simulink model "Math_transpose"  (R2017b)
settings: Solver=FixedStepDiscrete  StartTime=0.0  StopTime=10.0  FixedStep=0.200000  RelTol=1e-3  EnableMultiTasking=on
model workspace (MAT data in the model file):
  already_pp = 0
settings Model: Creator=ktrinh  LastModifiedBy=hbourbou
settings OptimizationCC: LifeSpan=inf
settings DebuggingCC: AlgebraicLoopMsg=error  ArtificialAlgebraicLoopMsg=error  SFUnexpectedBacktrackingDiag=warning  SFNoUnconditionalDefaultTransitionDiag=warning  SFExecutionAtInitializationDiag=none
settings HardwareCC: ProdBitPerSizeT=32  ProdBitPerPtrDiffT=32  ProdWordSize=32  ProdHWDeviceType=Specified
settings CodeAppCC: StateflowObjectComments=on
settings GRTTargetCC: TargetLangStandard=C89/C90 (ANSI)  GeneratePreprocessorConditionals=Disable all
settings ConfigComp: CovMetricSettings=dw  CovHtmlReporting=on  CovSaveCumulativeToWorkspaceVar=on  CovSaveSingleToWorkspaceVar=on  CovExternalEMLEnable=off

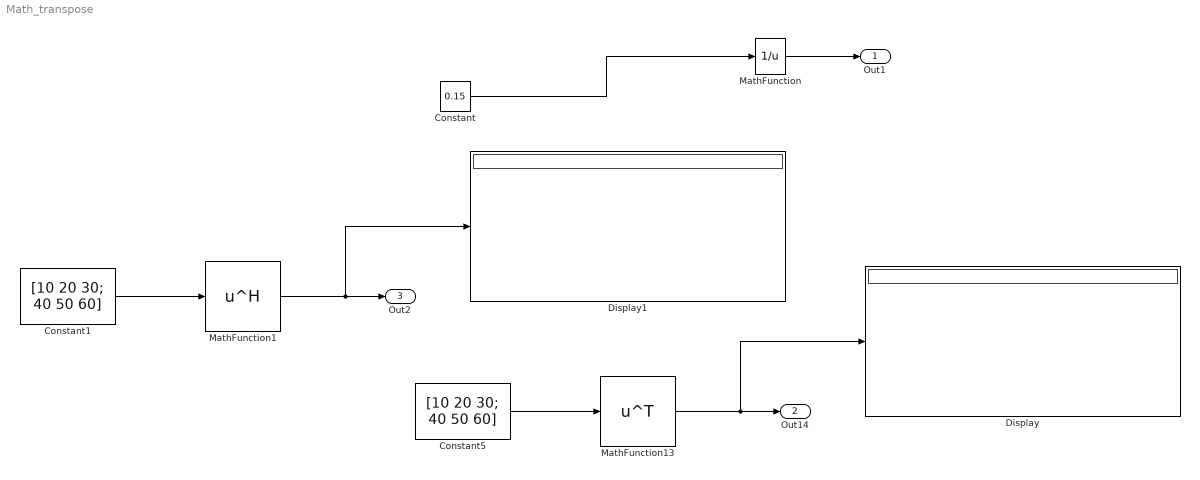
== system Math_transpose ==
  Constant : Constant  Value=0.15
  Constant1 : Constant  Value=[10 20 30; 40 50 60]
  Constant5 : Constant  Value=[10 20 30; 40 50 60]
  Display : Display
  Display1 : Display
  MathFunction : Math  Operator=reciprocal  SaturateOnIntegerOverflow=on
  MathFunction1 : Math  Operator=hermitian  SaturateOnIntegerOverflow=on
  MathFunction13 : Math  Operator=transpose  SaturateOnIntegerOverflow=on
  Out1 : Outport
  Out14 : Outport  Port=2
  Out2 : Outport  Port=3
  wires:
  MathFunction/1 -> Out1/1
  Constant/1 -> MathFunction/1
  MathFunction13/1 -> Display/1, Out14/1
  Constant5/1 -> MathFunction13/1
  MathFunction1/1 -> Display1/1, Out2/1
  Constant1/1 -> MathFunction1/1
